simulink model "a2"  (R2014b)
settings: Solver=ode45  StartTime=0.0  StopTime=10.0  RelTol=1e-3
settings Model: Creator=sigurd  LastModifiedBy=sigurd

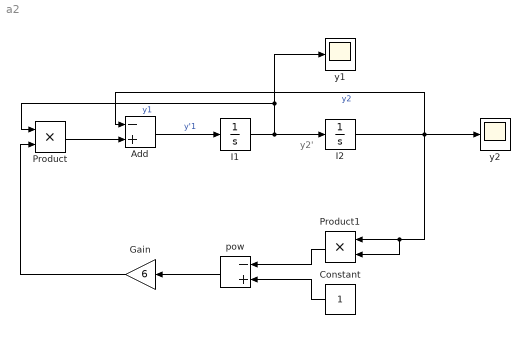
== system a2 ==
  note: y2'
  Add : Sum  Inputs=-+
  Constant : Constant
  Gain : Gain  Gain=6
  I1 : Integrator  InitialCondition=1  IgnoreLimit=on
  I2 : Integrator
  Product : Product
  Product1 : Product
  pow : Sum  Inputs=-+
  y1 : Scope
      settings: TimeRange=0.6400000000000006  YMin=0.6106818181818165  YMax=1.250681818181817
  y2 : Scope
  wires:
  Add/1 -> I1/1  "y'1"
  Product/1 -> Add/2
  pow/1 -> Gain/1
  I2/1 -> Add/1, Product1/1, Product1/2, y2/1  "y2"
  I1/1 -> y1/1, Product/1, I2/1  "y1"
  Product1/1 -> pow/1
  Constant/1 -> pow/2
  Gain/1 -> Product/2
